simulink model "NonLinearModelNorm"  (R2025b)
settings: Solver=ode1  StartTime=0.0  StopTime=120  FixedStep=0.001  RelTol=1e-3
values from neighbouring files (symbols this model uses):
  A_pade_IPS = [-407.436654315 1 0 0 -74702.0822758 0 1 0 -7101818.84366 0 0 1 ... (16 elements, 4x4)]    [pade_params.mat]
  A_pade_seg = [-1018.59163579 1 0 0 -466888.014224 0 1 0 -110965919.432 0 0 1 ... (16 elements, 4x4)]    [pade_params.mat]
  B_pade_IPS = [1 0 0 0]    [pade_params.mat]
  B_pade_seg = [1 0 0 0]    [pade_params.mat]
  C_pade_IPS = [-814.873308631 0 -14203637.6873 0]    [pade_params.mat]
  C_pade_seg = [-2037.18327158 0 -221931838.864 0]    [pade_params.mat]
  D_pade_IPS = 1    [pade_params.mat]
  D_pade_seg = 1    [pade_params.mat]
  du_ign_nom = -25    [Linearization.m]
  omega_e_nom = 100.43    [Linearization.m]
  p_m_nom = 23519.6    [Linearization.m]
  ratio_nom = 30.1967e-6    (= 3.01967e-05)    [Linearization.m]
  u_alpha_nom = 2    [Linearization.m]
undefined symbols (not defined in the file or in its folder): alpha0, alpha1, beta0, gamma0, gamma1, H_l, k_eta, kappa, lambda, nu0, nu1, R, sigma0, theta_e, Vc, Vd, Vm
settings Model: Creator=khanh  LastModifiedBy=khanh

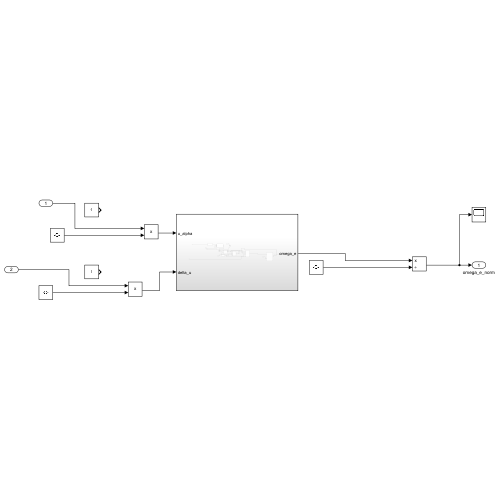
[thumbnail: Simulink's stored preview of the top-level diagram]
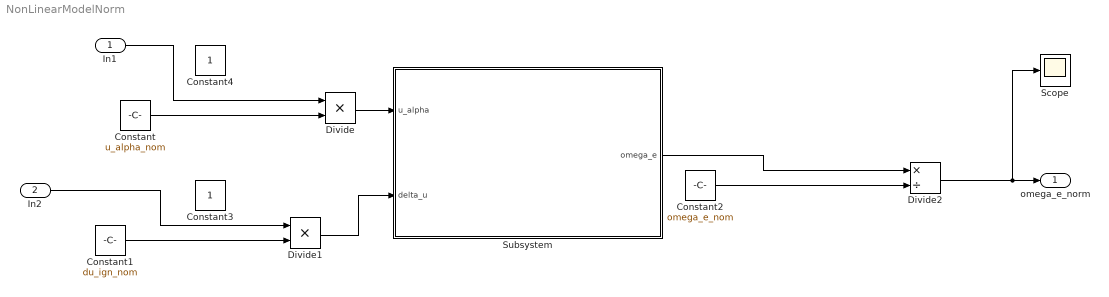
== system NonLinearModelNorm ==
  In1 : Inport
  In2 : Inport  Port=2
  Constant : Constant  Value=u_alpha_nom
  Constant1 : Constant  Value=du_ign_nom
  Constant2 : Constant  Value=omega_e_nom
  Constant3 : Constant
  Constant4 : Constant
  Divide : Product  Inputs=**
  Divide1 : Product  Inputs=**
  Divide2 : Product  Inputs=*/
  Scope : Scope
      settings: ActiveDisplayYMinimum=0.065232396712389534  ActiveDisplayYMaximum=1.4043452512553267
  Subsystem : Subsystem
  omega_e_norm : Outport
  wires:
  Constant/1 -> Divide/2
  Constant2/1 -> Divide2/2
  Subsystem/1(omega_e) -> Divide2/1
  Divide2/1 -> Scope/1, omega_e_norm/1
  Constant1/1 -> Divide1/2
  Divide/1 -> Subsystem/1(u_alpha)
  Divide1/1 -> Subsystem/2(delta_u)
  In1/1 -> Divide/1
  In2/1 -> Divide1/1

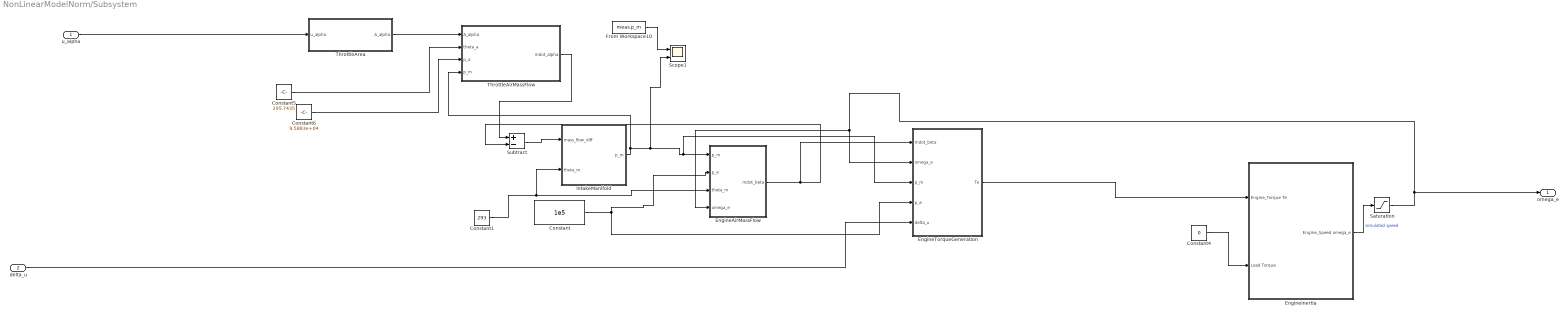
== system NonLinearModelNorm/Subsystem ==
  u_alpha : Inport
  delta_u : Inport  Port=2
  Constant : Constant  Value=1e5
  Constant1 : Constant  Value=293
  Constant4 : Constant  Value=0
  Constant5 : Constant  Value=295.7435
  Constant6 : Constant  Value=9.5883e+04
  EngineAirMassFlow : Subsystem
  EngineInertia : Subsystem
  EngineTorqueGeneration : Subsystem
  From Workspace10 : FromWorkspace  VariableName=meas.p_m
  IntakeManifold : Subsystem
  Saturation : Saturate  UpperLimit=500  LowerLimit=20
  Scope1 : Scope  NumInputPorts=2
      settings: ActiveDisplayYMinimum=-19631.671983717169  ActiveDisplayYMaximum=25125.259203208974  DataLoggingVariableName=ScopeData4
  Subtract : Sum  Inputs=+-
  ThrottleAirMassFlow : Subsystem
  ThrottleArea : Subsystem
  omega_e : Outport
  wires:
  Constant/1 -> EngineAirMassFlow/2(p_e), EngineTorqueGeneration/4(p_e)
  EngineInertia/1(Engine_Speed omega_e) -> Saturation/1  "simulated speed"
  IntakeManifold/1(p_m) -> ThrottleAirMassFlow/4(p_m), Scope1/2, EngineTorqueGeneration/3(p_m), EngineAirMassFlow/1(p_m)
  Constant6/1 -> ThrottleAirMassFlow/3(p_a)
  ThrottleAirMassFlow/1(mdot_alpha) -> Subtract/1
  Constant5/1 -> ThrottleAirMassFlow/2(theta_a)
  EngineAirMassFlow/1(mdot_beta) -> EngineTorqueGeneration/1(mdot_beta), Subtract/2
  delta_u/1 -> EngineTorqueGeneration/5(delta_u)
  From Workspace10/1 -> Scope1/1
  Subtract/1 -> IntakeManifold/1(mass_flow_diff)
  ThrottleArea/1(A_alpha) -> ThrottleAirMassFlow/1(A_alpha)
  Constant1/1 -> EngineAirMassFlow/3(theta_m), IntakeManifold/2(theta_m)
  EngineTorqueGeneration/1(Te) -> EngineInertia/1(Engine_Torque Te)
  u_alpha/1 -> ThrottleArea/1(u_alpha)
  Saturation/1 -> omega_e/1, EngineAirMassFlow/4(omega_e), EngineTorqueGeneration/2(omega_e)
  Constant4/1 -> EngineInertia/2(Load Torque)

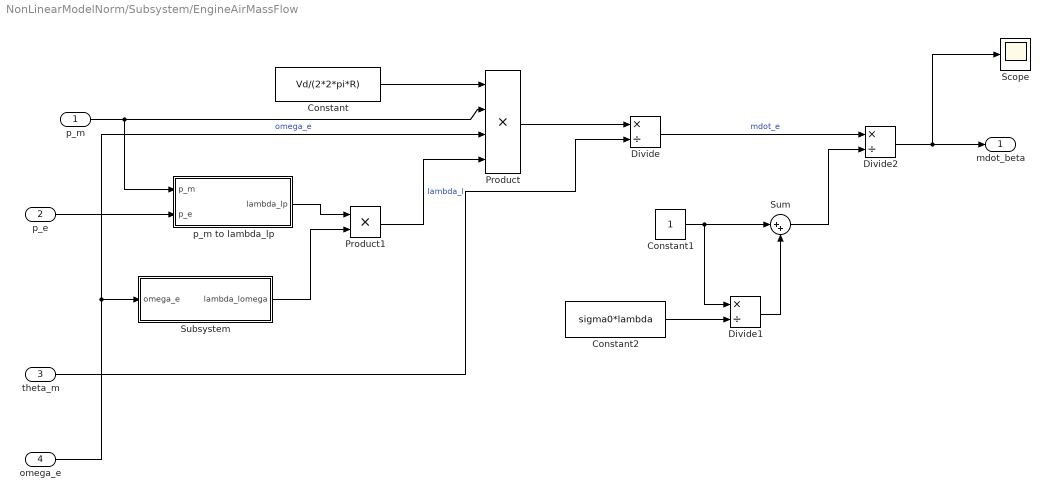
== system NonLinearModelNorm/Subsystem/EngineAirMassFlow ==
  p_m : Inport
  p_e : Inport  Port=2
  theta_m : Inport  Port=3
  omega_e : Inport  Port=4
  Constant : Constant  Value=Vd/(2*2*pi*R)
  Constant1 : Constant
  Constant2 : Constant  Value=sigma0*lambda
  Divide : Product  Inputs=*/
  Divide1 : Product  Inputs=*/
  Divide2 : Product  Inputs=*/
  Product : Product  Inputs=4
  Product1 : Product
  Scope : Scope
      settings: ActiveDisplayYMinimum=-1  ActiveDisplayYMaximum=1  DataLoggingVariableName=ScopeData3
  Subsystem : Subsystem
  Sum : Sum  Inputs=|++
  p_m to lambda_lp : Subsystem
  mdot_beta : Outport
  wires:
  Sum/1 -> Divide2/2
  Constant1/1 -> Divide1/1, Sum/1
  Divide/1 -> Divide2/1  "mdot_e"
  p_e/1 -> p_m to lambda_lp/2(p_e)
  Divide2/1 -> Scope/1, mdot_beta/1
  Constant/1 -> Product/1
  theta_m/1 -> Divide/2
  Product1/1 -> Product/4  "lambda_l"
  Constant2/1 -> Divide1/2
  omega_e/1 -> Product/3, Subsystem/1(omega_e)  "omega_e"
  Divide1/1 -> Sum/2
  p_m/1 -> p_m to lambda_lp/1(p_m), Product/2
  Product/1 -> Divide/1
  Subsystem/1(lambda_lomega) -> Product1/2
  p_m to lambda_lp/1(lambda_lp) -> Product1/1

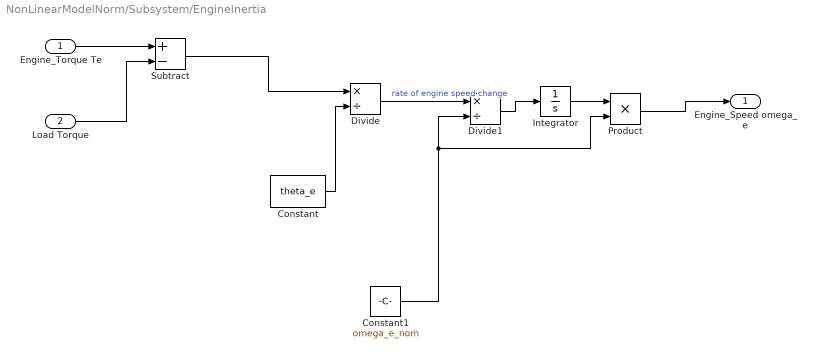
== system NonLinearModelNorm/Subsystem/EngineInertia ==
  Engine_Torque Te : Inport
  Load Torque : Inport  Port=2
  Constant : Constant  Value=theta_e
  Constant1 : Constant  Value=omega_e_nom
  Divide : Product  Inputs=*/
  Divide1 : Product  Inputs=*/
  Integrator : Integrator
  Product : Product
  Subtract : Sum  Inputs=+-
  Engine_Speed omega_e : Outport
  wires:
  Constant/1 -> Divide/2
  Divide/1 -> Divide1/1  "rate of engine speed change"
  Engine_Torque Te/1 -> Subtract/1
  Subtract/1 -> Divide/1
  Load Torque/1 -> Subtract/2
  Constant1/1 -> Product/2, Divide1/2
  Integrator/1 -> Product/1
  Product/1 -> Engine_Speed omega_e/1
  Divide1/1 -> Integrator/1

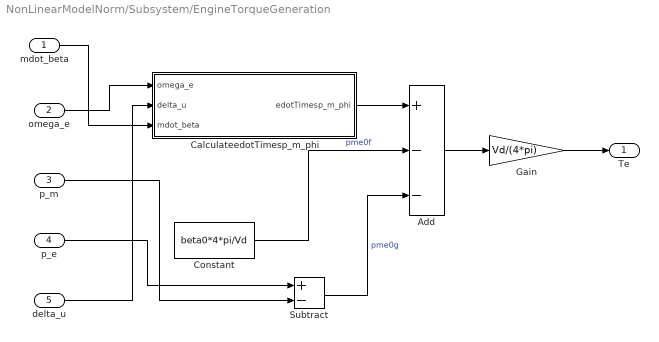
== system NonLinearModelNorm/Subsystem/EngineTorqueGeneration ==
  mdot_beta : Inport
  omega_e : Inport  Port=2
  p_m : Inport  Port=3
  p_e : Inport  Port=4
  delta_u : Inport  Port=5
  Add : Sum  Inputs=+--
  CalculateedotTimesp_m_phi : Subsystem
  Constant : Constant  Value=beta0*4*pi/Vd
  Gain : Gain  Gain=Vd/(4*pi)
  Subtract : Sum  Inputs=+-
  Te : Outport
  wires:
  Gain/1 -> Te/1
  Add/1 -> Gain/1
  Subtract/1 -> Add/3  "pme0g"
  p_m/1 -> Subtract/2
  delta_u/1 -> CalculateedotTimesp_m_phi/2(delta_u)
  CalculateedotTimesp_m_phi/1(edotTimesp_m_phi) -> Add/1
  mdot_beta/1 -> CalculateedotTimesp_m_phi/3(mdot_beta)
  Constant/1 -> Add/2  "pme0f"
  p_e/1 -> Subtract/1
  omega_e/1 -> CalculateedotTimesp_m_phi/1(omega_e)

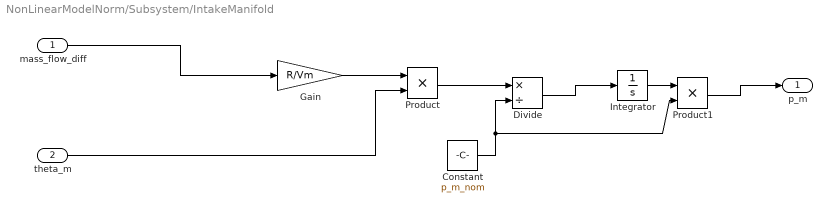
== system NonLinearModelNorm/Subsystem/IntakeManifold ==
  mass_flow_diff : Inport
  theta_m : Inport  Port=2
  Constant : Constant  Value=p_m_nom
  Divide : Product  Inputs=*/
  Gain : Gain  Gain=R/Vm
  Integrator : Integrator  InitialCondition=1
  Product : Product
  Product1 : Product
  p_m : Outport
  wires:
  Gain/1 -> Product/1
  theta_m/1 -> Product/2
  mass_flow_diff/1 -> Gain/1
  Product/1 -> Divide/1
  Divide/1 -> Integrator/1
  Constant/1 -> Product1/2, Divide/2
  Integrator/1 -> Product1/1
  Product1/1 -> p_m/1

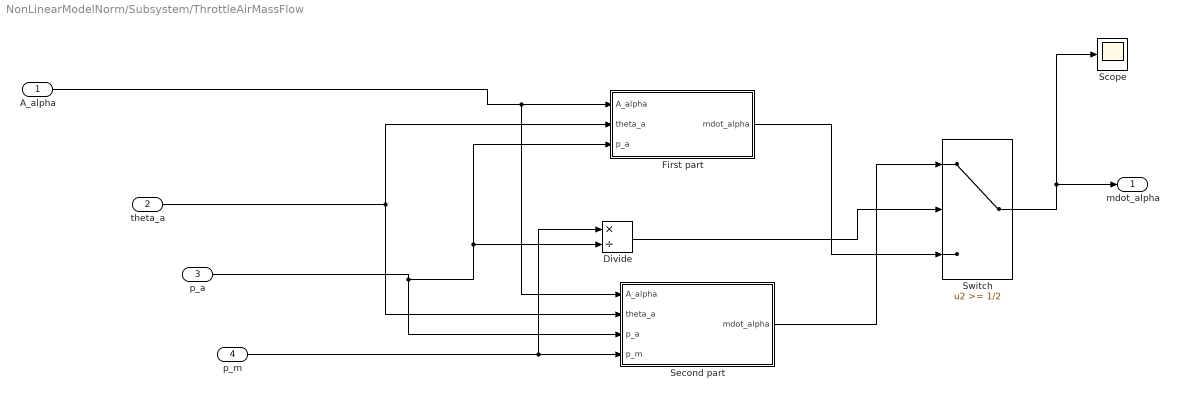
== system NonLinearModelNorm/Subsystem/ThrottleAirMassFlow ==
  A_alpha : Inport
  theta_a : Inport  Port=2
  p_a : Inport  Port=3
  p_m : Inport  Port=4
  Divide : Product  Inputs=*/
  First part : Subsystem
  Scope : Scope
      settings: ActiveDisplayYMinimum=-1  ActiveDisplayYMaximum=1
  "Second part " : Subsystem
  Switch : Switch  Threshold=1/2  SaturateOnIntegerOverflow=off  InputSameDT=off
  mdot_alpha : Outport
  wires:
  A_alpha/1 -> "Second part "/1(A_alpha), First part/1(A_alpha)
  p_a/1 -> "Second part "/3(p_a), First part/3(p_a), Divide/2
  p_m/1 -> "Second part "/4(p_m), Divide/1
  First part/1(mdot_alpha) -> Switch/3
  Switch/1 -> Scope/1, mdot_alpha/1
  Divide/1 -> Switch/2
  "Second part "/1(mdot_alpha) -> Switch/1
  theta_a/1 -> "Second part "/2(theta_a), First part/2(theta_a)

== system NonLinearModelNorm/Subsystem/ThrottleArea ==
  u_alpha : Inport
  Constant : Constant  Value=alpha0
  Gain : Gain  Gain=alpha1
  Sum : Sum  Inputs=|++
  A_alpha : Outport
  wires:
  Sum/1 -> A_alpha/1
  u_alpha/1 -> Gain/1
  Constant/1 -> Sum/2
  Gain/1 -> Sum/1

== system NonLinearModelNorm/Subsystem/EngineAirMassFlow/Subsystem ==
  omega_e : Inport
  Constant : Constant  Value=gamma0
  Gain : Gain  Gain=gamma1
  Sum : Sum  Inputs=|++
  lambda_lomega : Outport
  wires:
  Constant/1 -> Sum/1
  omega_e/1 -> Gain/1
  Gain/1 -> Sum/2
  Sum/1 -> lambda_lomega/1

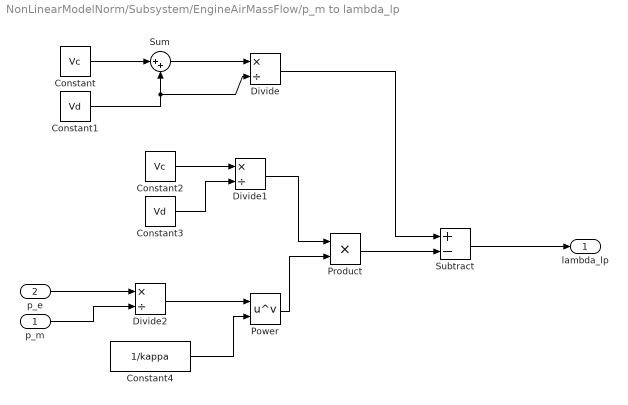
== system NonLinearModelNorm/Subsystem/EngineAirMassFlow/p_m to lambda_lp ==
  p_m : Inport
  p_e : Inport  Port=2
  Constant : Constant  Value=Vc
  Constant1 : Constant  Value=Vd
  Constant2 : Constant  Value=Vc
  Constant3 : Constant  Value=Vd
  Constant4 : Constant  Value=1/kappa
  Divide : Product  Inputs=*/
  Divide1 : Product  Inputs=*/
  Divide2 : Product  Inputs=*/
  Power : Math  Operator=pow
  Product : Product
  Subtract : Sum  Inputs=+-
  Sum : Sum  Inputs=|++
  lambda_lp : Outport
  wires:
  Constant/1 -> Sum/1
  Constant1/1 -> Sum/2, Divide/2
  Sum/1 -> Divide/1
  Constant2/1 -> Divide1/1
  Constant3/1 -> Divide1/2
  Divide2/1 -> Power/1
  Constant4/1 -> Power/2
  Divide1/1 -> Product/1
  Power/1 -> Product/2
  Divide/1 -> Subtract/1
  Product/1 -> Subtract/2
  Subtract/1 -> lambda_lp/1
  p_e/1 -> Divide2/1
  p_m/1 -> Divide2/2

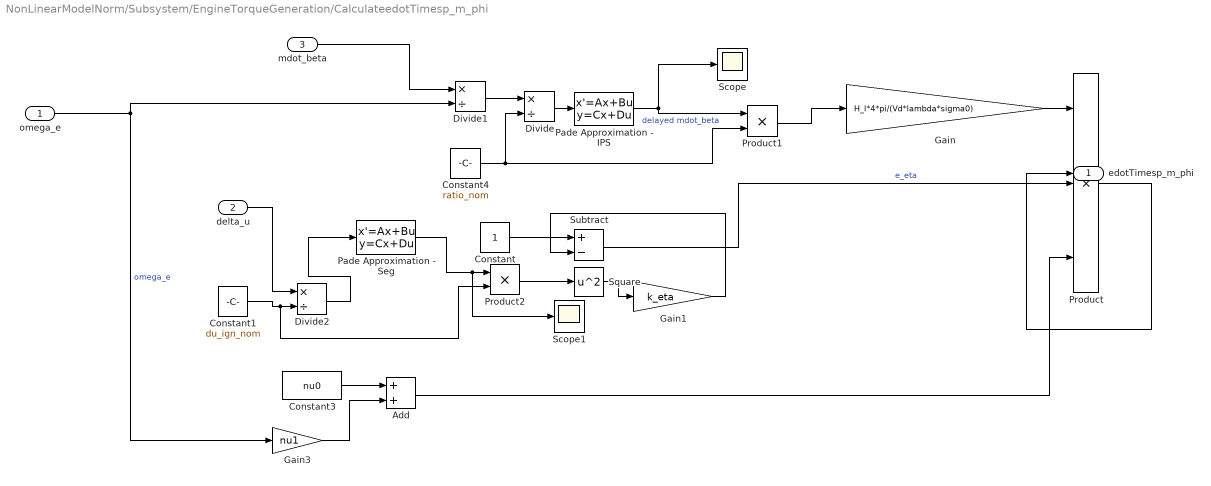
== system NonLinearModelNorm/Subsystem/EngineTorqueGeneration/CalculateedotTimesp_m_phi ==
  omega_e : Inport
  delta_u : Inport  Port=2
  mdot_beta : Inport  Port=3
  Add : Sum
  Constant : Constant
  Constant1 : Constant  Value=du_ign_nom
  Constant3 : Constant  Value=nu0
  Constant4 : Constant  Value=ratio_nom
  Divide : Product  Inputs=*/
  Divide1 : Product  Inputs=*/
  Divide2 : Product  Inputs=*/
  Gain : Gain  Gain=H_l*4*pi/(Vd*lambda*sigma0)
  Gain1 : Gain  Gain=k_eta
  Gain3 : Gain  Gain=nu1
  Pade Approximation - IPS : StateSpace  A=A_pade_IPS  B=B_pade_IPS  C=C_pade_IPS  D=D_pade_IPS  InitialCondition=-inv(A_pade_IPS)*B_pade_IPS
  Pade Approximation - Seg : StateSpace  A=A_pade_seg  B=B_pade_seg  C=C_pade_seg  D=D_pade_seg  InitialCondition=-inv(A_pade_seg)*B_pade_seg
  Product : Product  Inputs=3
  Product1 : Product
  Product2 : Product
  Scope : Scope
      settings: ActiveDisplayYMinimum=0.2313738795105974  ActiveDisplayYMaximum=4.1118173812597645  DataLoggingVariableName=ScopeData2
  Scope1 : Scope
      settings: ActiveDisplayYMinimum=-0.98423450737831819  ActiveDisplayYMaximum=3.6613440418684911  DataLoggingVariableName=ScopeData5
  Square : Math  Operator=square
  Subtract : Sum  Inputs=+-
  edotTimesp_m_phi : Outport
  wires:
  Constant/1 -> Subtract/1
  Gain1/1 -> Subtract/2
  Subtract/1 -> Product/2  "e_eta"
  omega_e/1 -> Gain3/1, Divide1/2  "omega_e"
  Constant3/1 -> Add/1
  Gain3/1 -> Add/2
  Gain/1 -> Product/1
  Add/1 -> Product/3
  Product/1 -> edotTimesp_m_phi/1
  mdot_beta/1 -> Divide1/1
  Square/1 -> Gain1/1
  Pade Approximation - IPS/1 -> Scope/1, Product1/1  "delayed mdot_beta"
  Pade Approximation - Seg/1 -> Scope1/1, Product2/1
  Divide1/1 -> Divide/1
  Divide/1 -> Pade Approximation - IPS/1
  Constant4/1 -> Product1/2, Divide/2
  Product1/1 -> Gain/1
  delta_u/1 -> Divide2/1
  Divide2/1 -> Pade Approximation - Seg/1
  Constant1/1 -> Product2/2, Divide2/2
  Product2/1 -> Square/1

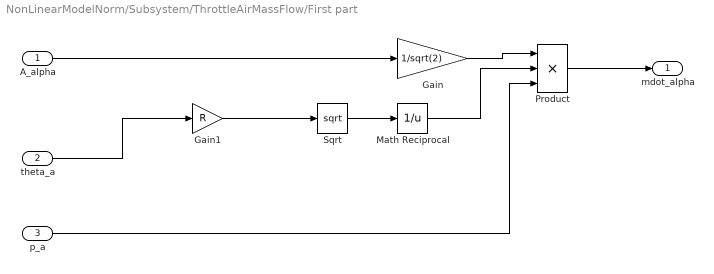
== system NonLinearModelNorm/Subsystem/ThrottleAirMassFlow/First part ==
  A_alpha : Inport
  theta_a : Inport  Port=2
  p_a : Inport  Port=3
  Gain : Gain  Gain=1/sqrt(2)
  Gain1 : Gain  Gain=R
  Math Reciprocal : Math  Operator=reciprocal  SignedPower=on
  Product : Product  Inputs=3
  Sqrt : Sqrt
  mdot_alpha : Outport
  wires:
  Sqrt/1 -> Math Reciprocal/1
  p_a/1 -> Product/3
  Gain/1 -> Product/1
  Gain1/1 -> Sqrt/1
  theta_a/1 -> Gain1/1
  Product/1 -> mdot_alpha/1
  A_alpha/1 -> Gain/1
  Math Reciprocal/1 -> Product/2

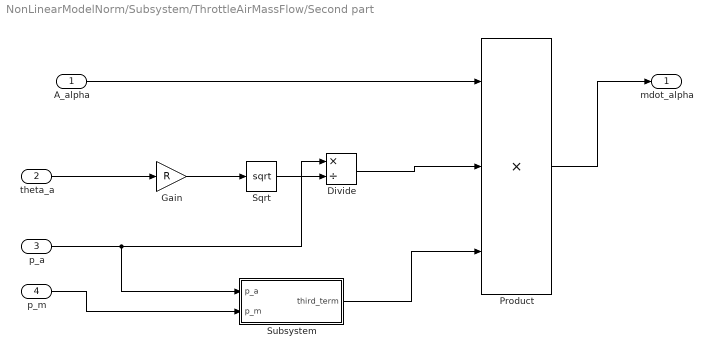
== system NonLinearModelNorm/Subsystem/ThrottleAirMassFlow/Second part  ==
  A_alpha : Inport
  theta_a : Inport  Port=2
  p_a : Inport  Port=3
  p_m : Inport  Port=4
  Divide : Product  Inputs=*/
  Gain : Gain  Gain=R
  Product : Product  Inputs=3
  Sqrt : Sqrt
  Subsystem : Subsystem
  mdot_alpha : Outport
  wires:
  Product/1 -> mdot_alpha/1
  A_alpha/1 -> Product/1
  theta_a/1 -> Gain/1
  Gain/1 -> Sqrt/1
  Sqrt/1 -> Divide/2
  p_a/1 -> Subsystem/1(p_a), Divide/1
  Divide/1 -> Product/2
  p_m/1 -> Subsystem/2(p_m)
  Subsystem/1(third_term) -> Product/3

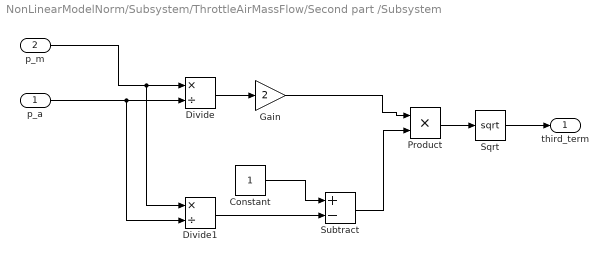
== system NonLinearModelNorm/Subsystem/ThrottleAirMassFlow/Second part /Subsystem ==
  p_a : Inport
  p_m : Inport  Port=2
  Constant : Constant
  Divide : Product  Inputs=*/
  Divide1 : Product  Inputs=*/
  Gain : Gain  Gain=2
  Product : Product
  Sqrt : Sqrt
  Subtract : Sum  Inputs=+-
  third_term : Outport
  wires:
  Divide/1 -> Gain/1
  p_a/1 -> Divide1/2, Divide/2
  p_m/1 -> Divide1/1, Divide/1
  Divide1/1 -> Subtract/2
  Constant/1 -> Subtract/1
  Gain/1 -> Product/1
  Subtract/1 -> Product/2
  Product/1 -> Sqrt/1
  Sqrt/1 -> third_term/1
